simulink model "ACC_RL_breach"  (R2021a)
settings: Solver=FixedStepAuto  StartTime=0.0  StopTime=T  RelTol=1e-3
undefined symbols (not defined in the file): amax_ego, amin_ego, D_default, t_gap, Ts, use_MPC, v0_ego, v0_lead, v_set, x0_ego, x0_lead
libraries: simulink x5, rllib x1
settings Model: OrderedModelArguments=off  Creator=The MathWorks, Inc.  LastModifiedBy=ldy
settings DataIOCC: ExternalInput=in_lead  ReturnWorkspaceOutputs=off
settings DebuggingCC: SFMachineParentedDataDiag=warning  ArithmeticOperatorsInVariantConditions=warning
settings SFSimCC: SimUseLocalCustomCode=off  CustomCodeUndefinedFunction=UseInterfaceOnly
settings RTWCC: RTWUseLocalCustomCode=off
settings CodeAppCC: StateflowObjectComments=on

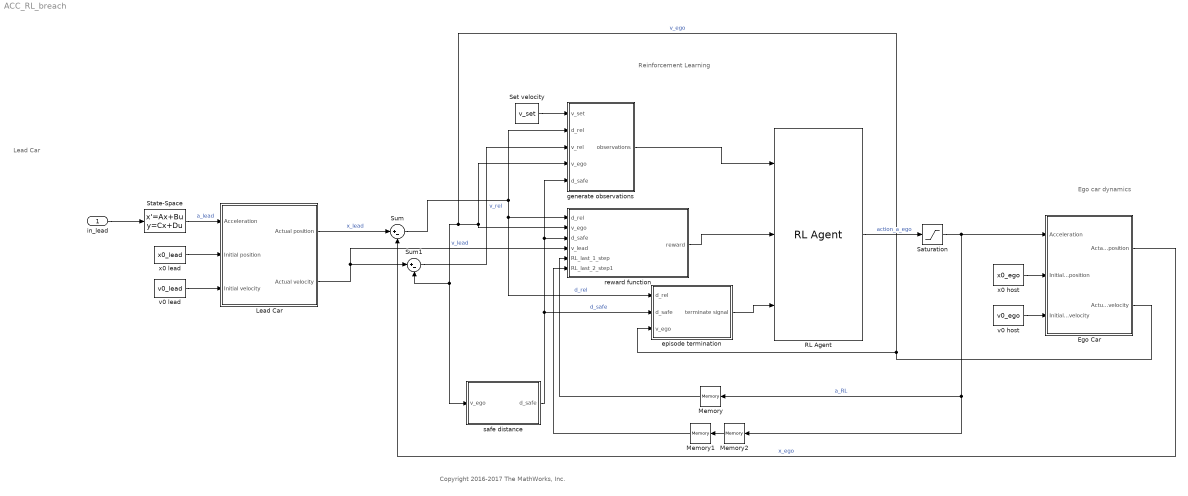
== system ACC_RL_breach ==
  note: Ego car dynamics
  note: Reinforcement Learning
  note: Lead Car
  note: Copyright 2016-2017 The MathWorks, Inc.
  in_lead : Inport
  Ego Car : Subsystem
  Lead Car : Subsystem
  Memory : Memory
  Memory1 : Memory
  Memory2 : Memory
  RL Agent : rllib/RL Agent  Agent=agent  ExternalActionAsInput=off  ProvideCumRwd=off  TreatAsDirectFeedthrough=on
  Saturation : Saturate  UpperLimit=amax_ego  LowerLimit=amin_ego
  Set velocity : Constant  Value=v_set  SampleTime=Ts
  State-Space : StateSpace  A=-10  B=10  D=0  InitialCondition=0
  Sum : Sum  Inputs=|+-
  Sum1 : Sum  Inputs=|+-
  episode termination : Subsystem
  generate observations : Subsystem
  reward function : Subsystem
  safe distance : Subsystem
  v0 host : Constant  Value=v0_ego  SampleTime=Ts
  v0 lead : Constant  Value=v0_lead  SampleTime=Ts
  x0 host : Constant  Value=x0_ego  SampleTime=Ts
  x0 lead : Constant  Value=x0_lead  SampleTime=Ts
  wires:
  x0 host/1 -> Ego Car/2(Initial position)
  Ego Car/1(Actaul position) -> Sum/2  "x_ego"
  Ego Car/2(Actual velocity) -> safe distance/1(v_ego), Sum1/2, reward function/2(v_ego), generate observations/4(v_ego), episode termination/3(v_ego)  "v_ego"
  v0 host/1 -> Ego Car/3(Initial velocity)
  Lead Car/1(Actual position) -> Sum/1  "x_lead"
  State-Space/1 -> Lead Car/1(Acceleration)  "a_lead"
  Lead Car/2(Actual velocity) -> Sum1/1, reward function/4(v_lead)  "v_lead"
  Sum/1 -> episode termination/1(d_rel), reward function/1(d_rel), generate observations/2(d_rel)  "d_rel"
  in_lead/1 -> State-Space/1
  safe distance/1(d_safe) -> reward function/3(d_safe), generate observations/5(d_safe), episode termination/2(d_safe)  "d_safe"
  Set velocity/1 -> generate observations/1(v_set)
  Sum1/1 -> generate observations/3(v_rel)  "v_rel"
  generate observations/1(observations) -> RL Agent/1
  reward function/1(reward) -> RL Agent/2
  episode termination/1(terminate signal) -> RL Agent/3
  RL Agent/1 -> Saturation/1  "action_a_ego"
  Saturation/1 -> Memory/1, Memory2/1, Ego Car/1(Acceleration)  "a_RL"
  Memory/1 -> reward function/5(RL_last_1_step)
  x0 lead/1 -> Lead Car/2(Initial position)
  v0 lead/1 -> Lead Car/3(Initial velocity)
  Memory2/1 -> Memory1/1
  Memory1/1 -> reward function/6(RL_last_2_step1)

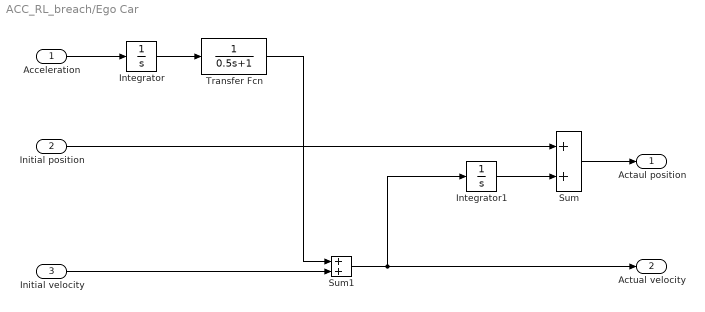
== system ACC_RL_breach/Ego Car ==
  Acceleration : Inport
  Initial position : Inport  Port=2
  Initial velocity : Inport  Port=3
  Integrator : Integrator
  Integrator1 : Integrator
  Sum : Sum
  Sum1 : Sum
  Transfer Fcn : TransferFcn  Denominator=[0.5 1]
  Actaul position : Outport  VectorParamsAs1DForOutWhenUnconnected=off
  Actual velocity : Outport  Port=2  VectorParamsAs1DForOutWhenUnconnected=off
  wires:
  Sum1/1 -> Integrator1/1, Actual velocity/1
  Initial velocity/1 -> Sum1/2
  Sum/1 -> Actaul position/1
  Transfer Fcn/1 -> Sum1/1
  Integrator/1 -> Transfer Fcn/1
  Acceleration/1 -> Integrator/1
  Initial position/1 -> Sum/1
  Integrator1/1 -> Sum/2

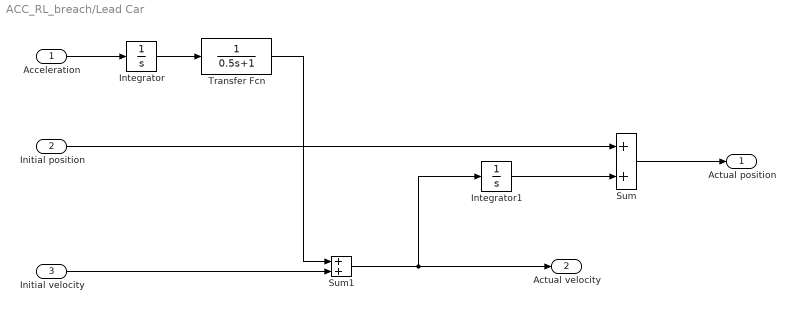
== system ACC_RL_breach/Lead Car ==
  Acceleration : Inport
  Initial position : Inport  Port=2
  Initial velocity : Inport  Port=3
  Integrator : Integrator
  Integrator1 : Integrator
  Sum : Sum
  Sum1 : Sum
  Transfer Fcn : TransferFcn  Denominator=[0.5 1]
  Actual position : Outport  VectorParamsAs1DForOutWhenUnconnected=off
  Actual velocity : Outport  Port=2  VectorParamsAs1DForOutWhenUnconnected=off
  wires:
  Transfer Fcn/1 -> Sum1/1
  Initial velocity/1 -> Sum1/2
  Sum/1 -> Actual position/1
  Integrator/1 -> Transfer Fcn/1
  Sum1/1 -> Integrator1/1, Actual velocity/1
  Acceleration/1 -> Integrator/1
  Initial position/1 -> Sum/1
  Integrator1/1 -> Sum/2

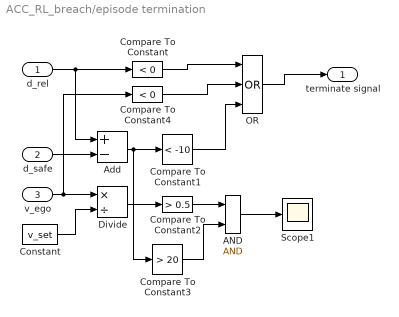
== system ACC_RL_breach/episode termination ==
  d_rel : Inport
  d_safe : Inport  Port=2
  v_ego : Inport  Port=3
  AND : Logic  IconShape=distinctive  AllPortsSameDT=off  OutDataTypeStr=boolean
  Add : Sum  Inputs=+-
  Compare To Constant : simulink/Logic and Bit Operations/Compare To Constant  relop=<  const=0  OutDataTypeStr=boolean
  Compare To Constant1 : simulink/Logic and Bit Operations/Compare To Constant  relop=<  const=-10  OutDataTypeStr=boolean
  Compare To Constant2 : simulink/Logic and Bit Operations/Compare To Constant  relop=>  const=0.5  OutDataTypeStr=boolean
  Compare To Constant3 : simulink/Logic and Bit Operations/Compare To Constant  relop=>  const=20  OutDataTypeStr=boolean
  Compare To Constant4 : simulink/Logic and Bit Operations/Compare To Constant  relop=<  const=0  OutDataTypeStr=boolean
  Constant : Constant  Value=v_set
  Divide : Product  Inputs=*/
  OR : Logic  Operator=OR  Inputs=3  IconShape=distinctive  AllPortsSameDT=off  OutDataTypeStr=boolean
  Scope1 : Scope
  terminate signal : Outport
  wires:
  d_rel/1 -> Compare To Constant/1, Add/1
  Compare To Constant1/1 -> OR/3
  Add/1 -> Compare To Constant1/1, Compare To Constant3/1
  d_safe/1 -> Add/2
  Constant/1 -> Divide/2
  v_ego/1 -> Compare To Constant4/1, Divide/1
  Divide/1 -> Compare To Constant2/1
  Compare To Constant2/1 -> AND/1
  AND/1 -> Scope1/1
  Compare To Constant3/1 -> AND/2
  OR/1 -> terminate signal/1
  Compare To Constant/1 -> OR/1
  Compare To Constant4/1 -> OR/2

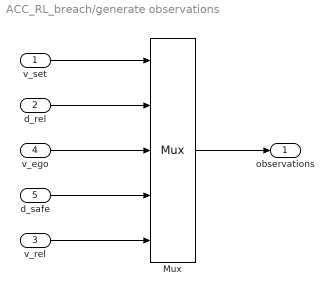
== system ACC_RL_breach/generate observations ==
  v_set : Inport
  d_rel : Inport  Port=2
  v_rel : Inport  Port=3
  v_ego : Inport  Port=4
  d_safe : Inport  Port=5
  Mux : Mux  Inputs=5
  observations : Outport
  wires:
  v_ego/1 -> Mux/3
  v_set/1 -> Mux/1
  Mux/1 -> observations/1
  d_safe/1 -> Mux/4
  v_rel/1 -> Mux/5
  d_rel/1 -> Mux/2

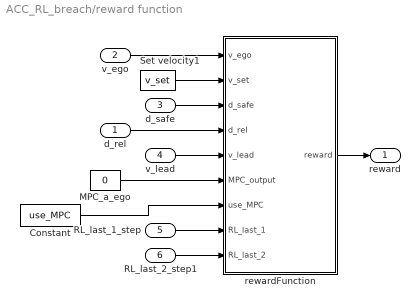
== system ACC_RL_breach/reward function ==
  d_rel : Inport
  v_ego : Inport  Port=2
  d_safe : Inport  Port=3
  v_lead : Inport  Port=4
  RL_last_1_step : Inport  Port=5
  RL_last_2_step1 : Inport  Port=6
  Constant : Constant  Value=use_MPC
  MPC_a_ego : Constant  Value=0
  Set velocity1 : Constant  Value=v_set  SampleTime=Ts
  rewardFunction : MATLAB Function  TreatAsAtomicUnit=on
  reward : Outport
  wires:
  Set velocity1/1 -> rewardFunction/2(v_set)
  d_rel/1 -> rewardFunction/4(d_rel)
  v_ego/1 -> rewardFunction/1(v_ego)
  rewardFunction/1(reward) -> reward/1
  d_safe/1 -> rewardFunction/3(d_safe)
  v_lead/1 -> rewardFunction/5(v_lead)
  Constant/1 -> rewardFunction/7(use_MPC)
  RL_last_1_step/1 -> rewardFunction/8(RL_last_1)
  RL_last_2_step1/1 -> rewardFunction/9(RL_last_2)
  MPC_a_ego/1 -> rewardFunction/6(MPC_output)

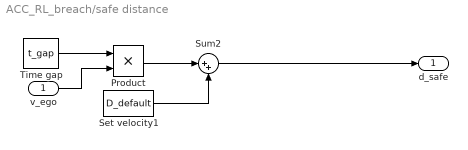
== system ACC_RL_breach/safe distance ==
  v_ego : Inport
  Product : Product
  Set velocity1 : Constant  Value=D_default  SampleTime=Ts
  Sum2 : Sum  Inputs=|++
  Time gap : Constant  Value=t_gap  SampleTime=Ts
  d_safe : Outport
  wires:
  Time gap/1 -> Product/1
  Sum2/1 -> d_safe/1
  v_ego/1 -> Product/2
  Product/1 -> Sum2/1
  Set velocity1/1 -> Sum2/2

== matlab function ACC_RL_breach/reward function/rewardFunction ==
  data: v_ego input; reward output; v_set input; d_safe input; d_rel input; v_lead input; MPC_output input; use_MPC input; RL_last_1 input; RL_last_2 input
function reward = fcn(v_ego, v_set, d_safe, d_rel, v_lead, MPC_output, use_MPC, RL_last_1, RL_last_2)
% 
% % case 1: negative reward if d_rel < d_safe
% if d_rel < d_safe 
%     reward = -tanh((d_safe - d_rel)/5);
% 
% % case 2: negative reward for v_ego beyond v_set
% elseif v_ego > v_set
%     v_error = v_ego-v_set;
%     reward = -tanh(v_error/2);
%     
% % case 4: positive reward for v_ego appraoching to v_set
% elseif  d_rel - d_safe <=2
%     v_error = v_ego - v_lead;
%     reward = exp(-(v_error/3)^2);
% else 
% %     v_error = v_ego-min([v_set,v_lead]);
%     v_error = v_ego - v_set;
%     reward = exp(-(v_error/3)^2);
%     
% end
d_reward = 0;
v_reward = 0;

% negative reward for safe distance violation
if d_rel < d_safe +0.25
    d_reward = -tanh((d_safe+0.25 - d_rel)/5);
end

% negative reward for user-set velocity violation
if v_ego > v_set
    v_error = v_ego-v_set;
    v_reward = -tanh(v_error/2);
end

% the positive potential reward is based on the error velocity between v_set and v_ego
if d_rel - d_safe < 0.5
    v_error = v_ego - min(v_set, v_lead);
else
    v_error = v_ego - v_set;
end

a_ego_erro = abs(RL_last_1 - RL_last_2);

RL_reward = exp(-(v_error/3)^2) + d_reward + v_reward - 0.1*tanh(a_ego_erro/1.5) - (RL_last_1/10)^2; 
% RL_reward = exp(-(v_error/3)^2) + d_reward + v_reward; 

if RL_reward < 0
    reward = RL_reward;
elseif use_MPC
    MPC_reward = exp(-(MPC_output - RL_last_1)^2);
    reward = RL_reward*0.8 + MPC_reward*0.2;
else
    reward = RL_reward;
end
